simulink model "modeling_thermostat"  (R2022b)
settings: Solver=VariableStepAuto  StartTime=0.0  StopTime=10.0  RelTol=1e-3
undefined symbols (not defined in the file): Ki, Kp, Ts
settings Model: Creator=Haina Bhawnani  LastModifiedBy=Haina Bhawnani

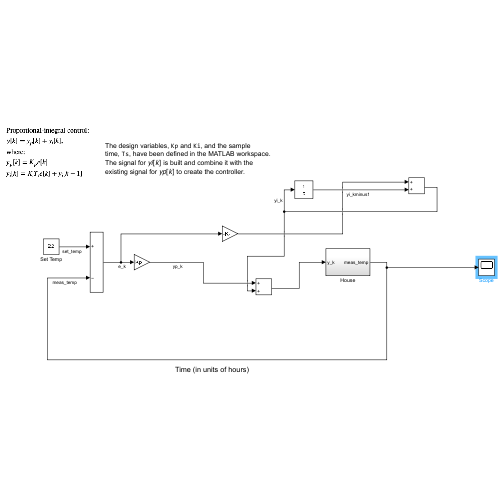
[thumbnail: Simulink's stored preview of the top-level diagram]
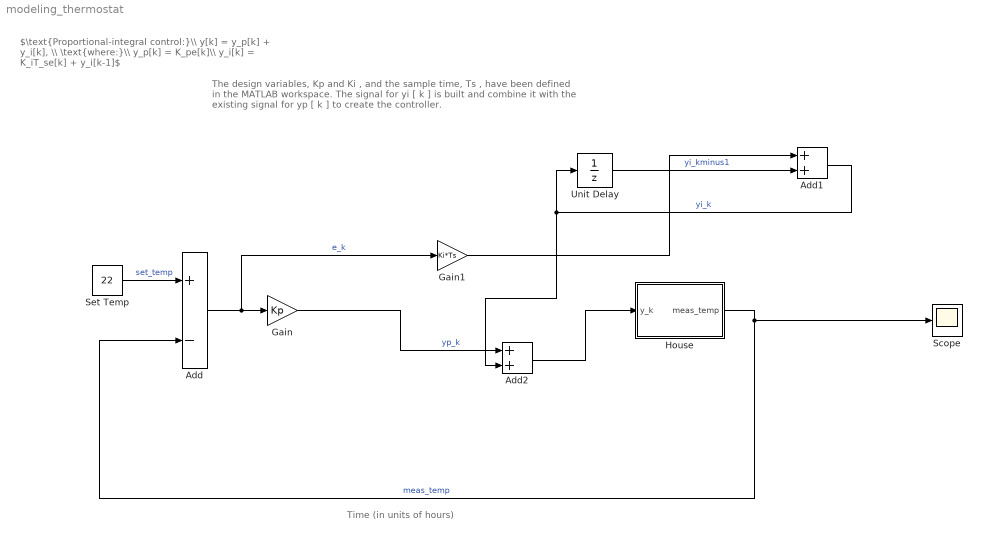
== system modeling_thermostat ==
  note: The design variables, Kp and Ki , and the sample time, Ts , have been defined in the MATLAB workspace.
      | The signal for yi [ k ] is built and combine it with the existing signal for yp [ k ] to create the controller.
  note: $\text{Proportional-integral control:}\\ y[k] = y_p[k] + y_i[k], \\ \text{where:}\\ y_p[k] = K_pe[k]\\ y_i[k] = K_iT_se[k] + y_i[k-1]$
  note: Time (in units of hours)
  Add : Sum  Inputs=+-
  Add1 : Sum
  Add2 : Sum
  Gain : Gain  Gain=Kp
  Gain1 : Gain  Gain=Ki*Ts
  House : Subsystem
  Scope : Scope
  Set Temp : Constant  Value=22
  Unit Delay : UnitDelay  SampleTime=Ts  HasFrameUpgradeWarning=on
  wires:
  Unit Delay/1 -> Add1/2  "yi_kminus1"
  Add1/1 -> Add2/2, Unit Delay/1  "yi_k"
  Gain/1 -> Add2/1  "yp_k"
  Set Temp/1 -> Add/1  "set_temp"
  Add/1 -> Gain1/1, Gain/1  "e_k"
  Gain1/1 -> Add1/1
  House/1(meas_temp) -> Scope/1, Add/2  "meas_temp"
  Add2/1 -> House/1(y_k)

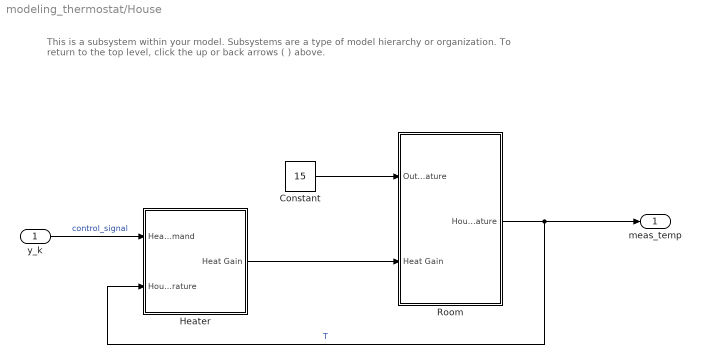
== system modeling_thermostat/House ==
  note: This is a subsystem within your model. Subsystems are a type of model hierarchy or organization.
      |
      | To return to the top level, click the up or back arrows ( ) above.
  y_k : Inport
  Constant : Constant  Value=15
  Heater : Subsystem
  Room : Subsystem
  meas_temp : Outport  VectorParamsAs1DForOutWhenUnconnected=off
  wires:
  y_k/1 -> Heater/1(Heater Command)  "control_signal"
  Heater/1(Heat Gain) -> Room/2("Heat Gain ")
  Room/1(House Temperature) -> meas_temp/1, Heater/2(House Temperature)  "T"
  Constant/1 -> Room/1(Outside Temperature)

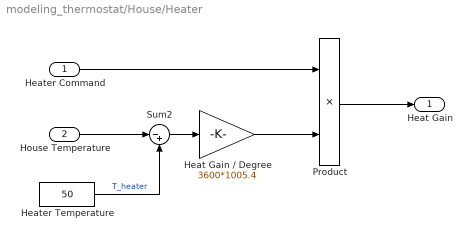
== system modeling_thermostat/House/Heater ==
  Heater Command : Inport
  House Temperature : Inport  Port=2
  Heat Gain / Degree : Gain  Gain=3600*1005.4
  Heater Temperature : Constant  Value=50
  Product : Product  RndMeth=Zero
  Sum2 : Sum  Inputs=|-+
  Heat Gain : Outport  Unit=joule/hour  VectorParamsAs1DForOutWhenUnconnected=off
  wires:
  Product/1 -> Heat Gain/1
  Heater Command/1 -> Product/1
  Heat Gain / Degree/1 -> Product/2
  Sum2/1 -> Heat Gain / Degree/1
  House Temperature/1 -> Sum2/1
  Heater Temperature/1 -> Sum2/2  "T_heater"

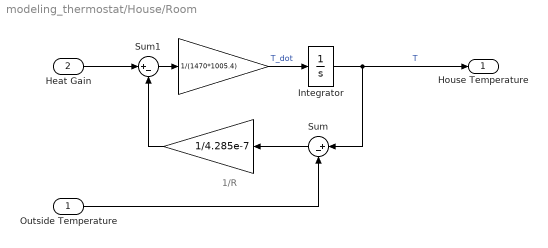
== system modeling_thermostat/House/Room ==
  note: 1/R
  Outside Temperature : Inport  Unit=°C
  "Heat Gain " : Inport  Port=2  Unit=joule/h
  " " : Gain  Gain=1/4.285e-7  SaturateOnIntegerOverflow=on  OutDataTypeStr=Inherit: Same as input  ParamDataTypeStr=Inherit: Same as input
  "  " : Gain  Gain=1/(1470*1005.4)  SaturateOnIntegerOverflow=on  OutDataTypeStr=Inherit: Same as input  ParamDataTypeStr=Inherit: Same as input
  Integrator : Integrator
  Sum : Sum  Inputs=|+-
  Sum1 : Sum  Inputs=|+-  InputSameDT=on  SaturateOnIntegerOverflow=on  OutDataTypeStr=Inherit: Same as first input
  House Temperature : Outport  Unit=°C  VectorParamsAs1DForOutWhenUnconnected=off
  wires:
  Outside Temperature/1 -> Sum/2
  Sum/1 -> " "/1
  " "/1 -> Sum1/2
  Integrator/1 -> House Temperature/1, Sum/1  "T"
  "  "/1 -> Integrator/1  "T_dot"
  Sum1/1 -> "  "/1
  "Heat Gain "/1 -> Sum1/1
